simulink subsystem "LRLM_ECU"  (R2021a)
settings: Solver=VariableStepAuto  StartTime=0.0  StopTime=10.0  RelTol=1e-3
values from neighbouring files (symbols this model uses):
  op_type = 2    [baseworkspace_variables.mat]
libraries: LRLM x4, simulink x2, pil_lib x1, BCM x1
settings Model: Creator=Sai229  LastModifiedBy=Sai229

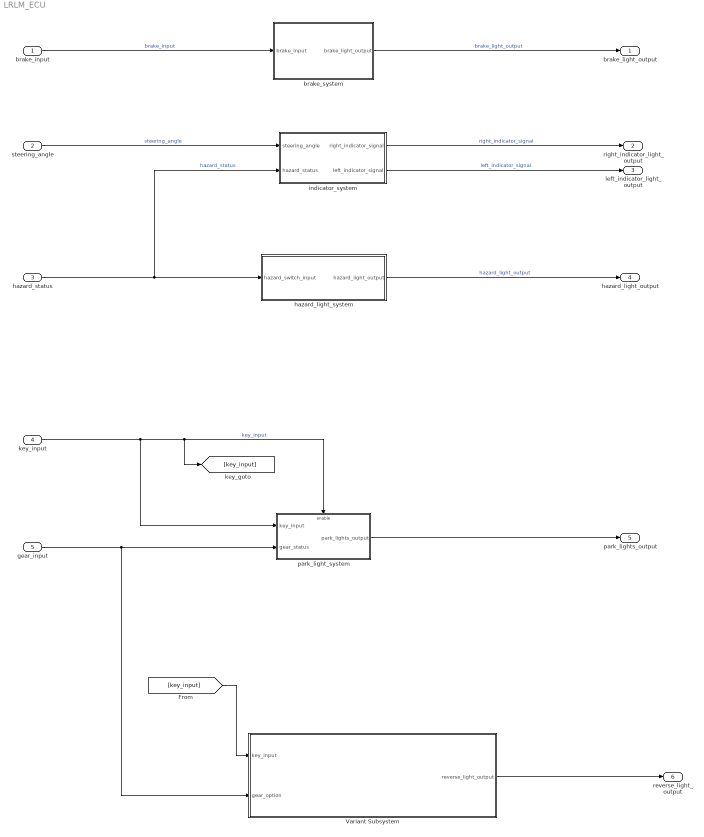
== system LRLM_ECU ==
  brake_input : Inport
  steering_angle : Inport  Port=2
  hazard_status : Inport  Port=3
  key_input : Inport  Port=4
  gear_input : Inport  Port=5
  Variant Subsystem : Subsystem  Variant=on
  brake_system : Subsystem  TreatAsAtomicUnit=on
      mask Display: disp("Brake System");
  hazard_light_system : Subsystem
  indicator_system : Subsystem  TreatAsAtomicUnit=on
  park_light_system : Subsystem
  brake_light_output : Outport
  right_indicator_light_output : Outport  Port=2
  left_indicator_light_output : Outport  Port=3
  hazard_light_output : Outport  Port=4
  park_lights_output : Outport  Port=5
  reverse_light_output : Outport  Port=6
  wires:
  hazard_light_system/1(hazard_light_output) -> hazard_light_output/1  "hazard_light_output"
  brake_input/1 -> brake_system/1(brake_input)  "brake_input"
  park_light_system/1(park_lights_output) -> park_lights_output/1
  key_input/1 -> park_light_system/Enable, [key_input], park_light_system/1(key_input)  "key_input"
  hazard_status/1 -> hazard_light_system/1(hazard_switch_input), indicator_system/2(hazard_status)  "hazard_status"
  indicator_system/2(left_indicator_signal) -> left_indicator_light_output/1  "left_indicator_signal"
  indicator_system/1(right_indicator_signal) -> right_indicator_light_output/1  "right_indicator_signal"
  steering_angle/1 -> indicator_system/1(steering_angle)  "steering_angle"
  brake_system/1(brake_light_output) -> brake_light_output/1  "brake_light_output"
  gear_input/1 -> park_light_system/2(gear_status), Variant Subsystem/2(gear_option)
  [key_input] -> Variant Subsystem/1(key_input)
  Variant Subsystem/1(reverse_light_output) -> reverse_light_output/1

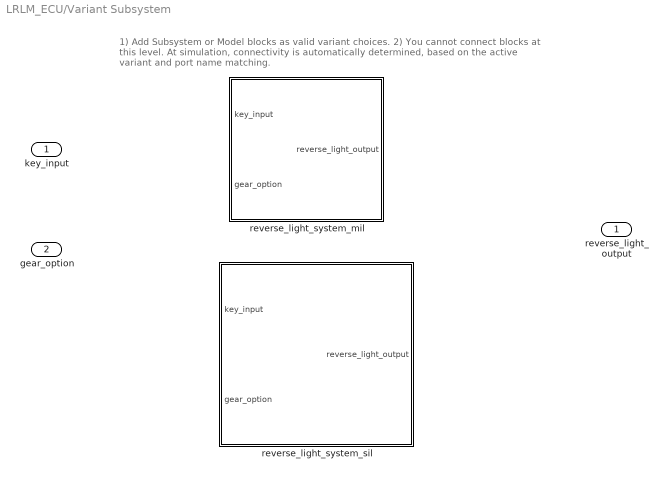
== system LRLM_ECU/Variant Subsystem ==
  note: 1) Add Subsystem or Model blocks as valid variant choices.
      | 2) You cannot connect blocks at this level. At simulation, connectivity is automatically
      | determined, based on the active variant and port name matching.
  key_input : Inport
  gear_option : Inport  Port=2
  reverse_light_system_mil : Subsystem  TreatAsAtomicUnit=on  VariantControl=reverse_light_sys_sil  mask{out_type=Reverse Lights will not Blink}
      mask prompts: out_type "Output type"
      mask init:
      | assignin('base','op_type',out_type);
      mask TypeOptions out_type: Reverse Lights will Blink | Reverse Lights will not Blink
  reverse_light_system_sil : Subsystem  DialogController=pil_create_dialog  LoadFcn=|  VariantControl=reverse_light_sys_mil
      | try
      |    if ~strcmp(rtw.pil.getPILVersion, '9.10 (R2021a)_15')
      |       set_param(gcb, 'DialogController', '');
      |       set_param(gcb, 'DialogControllerArgs', '');
      |    end
      | catch e
      |       set_param(gcb, 'DialogController', '');
      |       set_param(gcb, 'DialogControllerArgs', '');
      | end
      mask help: PIL:pil:XILBlockMaskDesc
      mask Display: disp('SIL');
  reverse_light_output : Outport

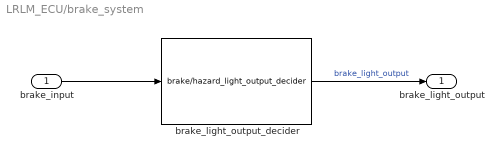
== system LRLM_ECU/brake_system ==
  brake_input : Inport
  brake_light_output_decider : LRLM/brake//hazard_light_output_decider
      settings: SourceProductName=LRLM Library
  brake_light_output : Outport
  wires:
  brake_light_output_decider/1 -> brake_light_output/1  "brake_light_output"
  brake_input/1 -> brake_light_output_decider/1

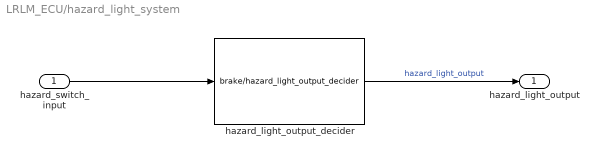
== system LRLM_ECU/hazard_light_system ==
  hazard_switch_input : Inport
  hazard_light_output_decider : LRLM/brake//hazard_light_output_decider
      settings: SourceProductName=LRLM Library
  hazard_light_output : Outport
  wires:
  hazard_light_output_decider/1 -> hazard_light_output/1  "hazard_light_output"
  hazard_switch_input/1 -> hazard_light_output_decider/1

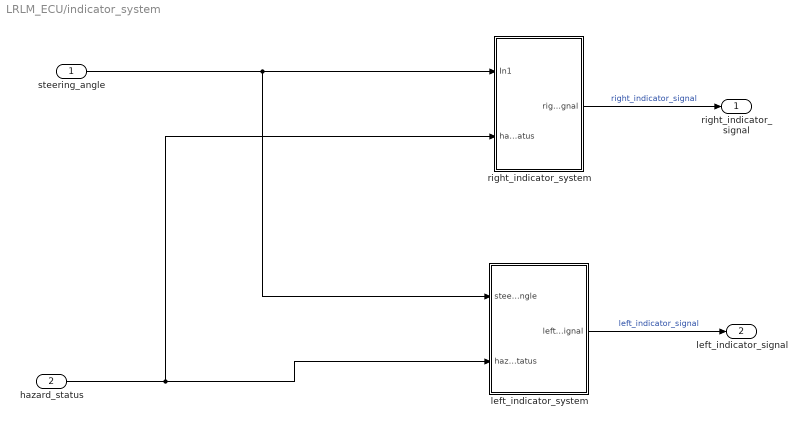
== system LRLM_ECU/indicator_system ==
  steering_angle : Inport
  hazard_status : Inport  Port=2
  left_indicator_system : Subsystem
  right_indicator_system : Subsystem
  right_indicator_signal : Outport
  left_indicator_signal : Outport  Port=2
  wires:
  steering_angle/1 -> right_indicator_system/1(In1), left_indicator_system/1(steering_angle)
  hazard_status/1 -> left_indicator_system/2(hazard_status), right_indicator_system/2(hazard_status)
  right_indicator_system/1(right_indicator_signal) -> right_indicator_signal/1  "right_indicator_signal"
  left_indicator_system/1(left_indicator_signal) -> left_indicator_signal/1  "left_indicator_signal"

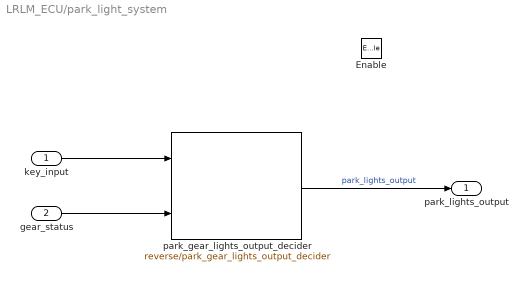
== system LRLM_ECU/park_light_system ==
  key_input : Inport
  gear_status : Inport  Port=2
  Enable : EnablePort  StatesWhenEnabling=reset
  park_gear_lights_output_decider : BCM/reverse//park_gear_lights_output_decider  gear_option=Park
      settings: SourceProductName=BCM Library
  park_lights_output : Outport
  wires:
  park_gear_lights_output_decider/1 -> park_lights_output/1  "park_lights_output"
  gear_status/1 -> park_gear_lights_output_decider/2
  key_input/1 -> park_gear_lights_output_decider/1

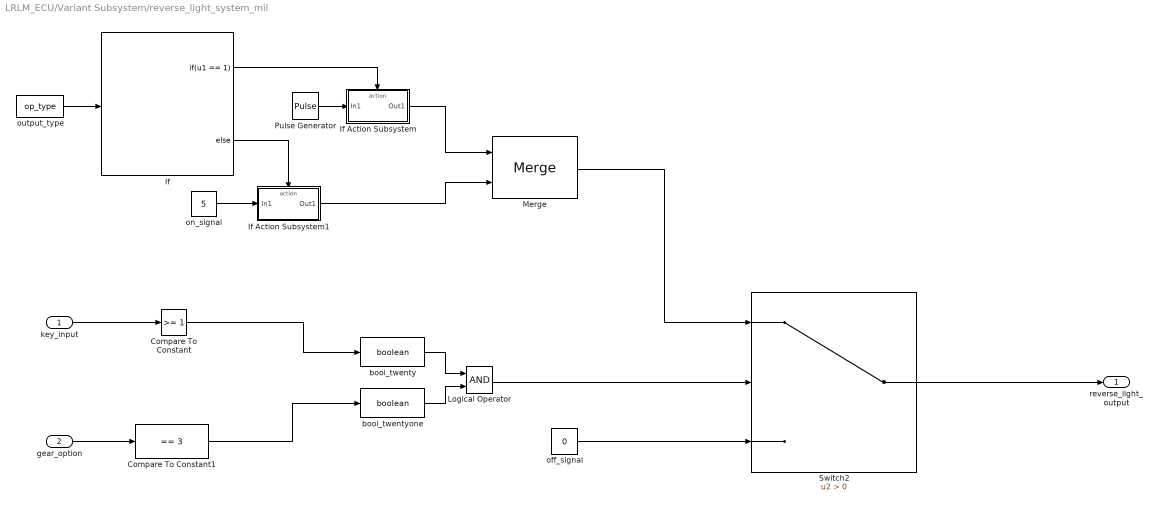
== system LRLM_ECU/Variant Subsystem/reverse_light_system_mil ==
  key_input : Inport
  gear_option : Inport  Port=2
  Compare To Constant : simulink/Logic and Bit Operations/Compare To Constant  relop=>=  const=1  OutDataTypeStr=boolean
  Compare To Constant1 : simulink/Logic and Bit Operations/Compare To Constant  relop===  const=3  OutDataTypeStr=boolean
  If : If  IfExpression=u1 == 1
  If Action Subsystem : Subsystem  TreatAsAtomicUnit=on
  If Action Subsystem1 : Subsystem  TreatAsAtomicUnit=on
  Logical Operator : Logic  AllPortsSameDT=off  OutDataTypeStr=boolean
  Merge : Merge
  Pulse Generator : DiscretePulseGenerator  PulseType=Time based  Amplitude=5  Period=0.1  PulseWidth=5
  Switch2 : Switch  Criteria=u2 > Threshold
  bool_twenty : DataTypeConversion  OutDataTypeStr=boolean
  bool_twentyone : DataTypeConversion  OutDataTypeStr=boolean
  off_signal : Constant  Value=0
  on_signal : Constant  Value=5
  output_type : Constant  Value=op_type
  reverse_light_output : Outport
  wires:
  Switch2/1 -> reverse_light_output/1
  output_type/1 -> If/1
  on_signal/1 -> If Action Subsystem1/1(In1)
  Pulse Generator/1 -> If Action Subsystem/1(In1)
  If/2 -> If Action Subsystem1/Action
  If Action Subsystem1/1(Out1) -> Merge/2
  If/1 -> If Action Subsystem/Action
  If Action Subsystem/1(Out1) -> Merge/1
  key_input/1 -> Compare To Constant/1
  gear_option/1 -> Compare To Constant1/1
  Compare To Constant1/1 -> bool_twentyone/1
  Compare To Constant/1 -> bool_twenty/1
  bool_twenty/1 -> Logical Operator/1
  Merge/1 -> Switch2/1
  off_signal/1 -> Switch2/3
  bool_twentyone/1 -> Logical Operator/2
  Logical Operator/1 -> Switch2/2

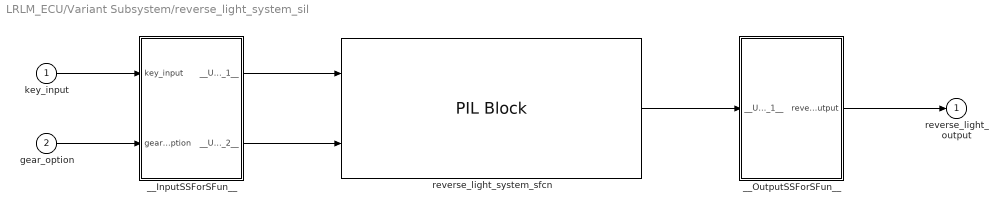
== system LRLM_ECU/Variant Subsystem/reverse_light_system_sil ==
  key_input : Inport
  gear_option : Inport  Port=2
  __InputSSForSFun__ : Subsystem
  __OutputSSForSFun__ : Subsystem
  reverse_light_system_sfcn : pil_lib/PIL Block  SimulationMode=SIL  IsTopModelPIL=off  CodeDir=D:\Genesis\HILClimbers_Public_Project\reverse_light_system_ert_rtw  AnchorDir=D:\Genesis\HILClimbers_Public_Project  ConfigName=Software-in-the-Loop (SIL)  XrelIsTopModelCode=on  XrelIsReusable=off  XrelDWorkNames={}  XrelDWorkTypes={}  XrelModelArgVals={}  XrelOrderedParamNames={}
      settings: SourceProductBaseCode=RT
  reverse_light_output : Outport
  wires:
  __OutputSSForSFun__/1(reverse_light_output) -> reverse_light_output/1
  reverse_light_system_sfcn/1 -> __OutputSSForSFun__/1(__UniqueInportName__1__)
  __InputSSForSFun__/2(__UniqueOutportName__2__) -> reverse_light_system_sfcn/2
  __InputSSForSFun__/1(__UniqueOutportName__1__) -> reverse_light_system_sfcn/1
  gear_option/1 -> __InputSSForSFun__/2(gear_option)
  key_input/1 -> __InputSSForSFun__/1(key_input)

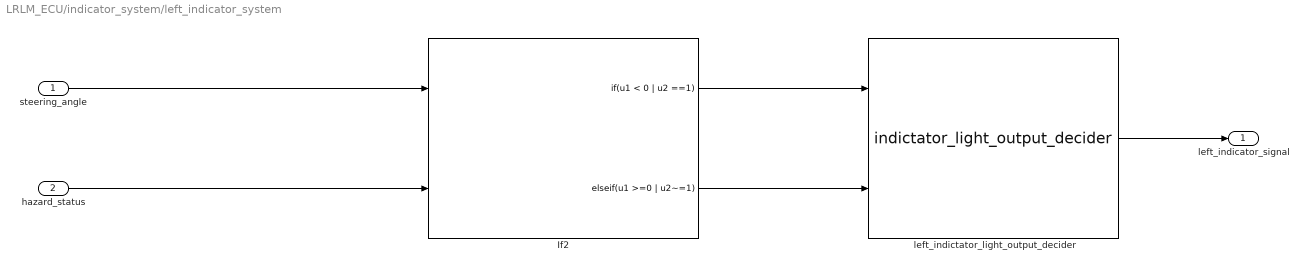
== system LRLM_ECU/indicator_system/left_indicator_system ==
  steering_angle : Inport
  hazard_status : Inport  Port=2
  If2 : If  NumInputs=2  IfExpression=u1 < 0 | u2 ==1  ElseIfExpressions=u1 >=0 | u2~=1  ShowElse=off
  left_indictator_light_output_decider : LRLM/indictator_light_output_decider
      settings: SourceProductName=LRLM Library
  left_indicator_signal : Outport
  wires:
  left_indictator_light_output_decider/1 -> left_indicator_signal/1
  If2/2 -> left_indictator_light_output_decider/2
  If2/1 -> left_indictator_light_output_decider/1
  steering_angle/1 -> If2/1
  hazard_status/1 -> If2/2

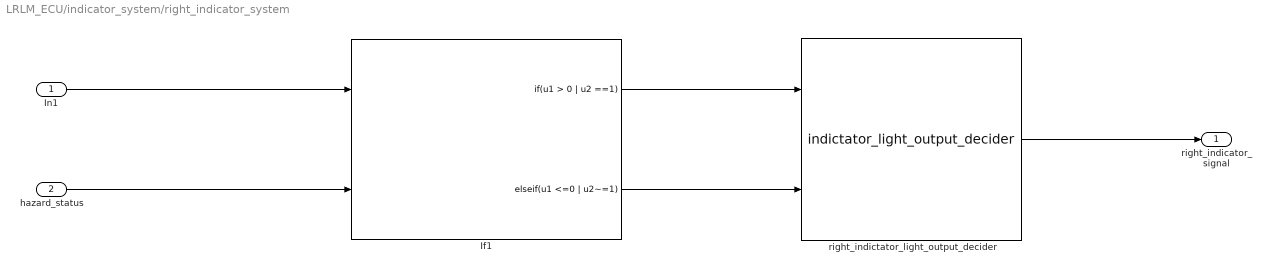
== system LRLM_ECU/indicator_system/right_indicator_system ==
  In1 : Inport
  hazard_status : Inport  Port=2
  If1 : If  NumInputs=2  IfExpression=u1 > 0 | u2 ==1  ElseIfExpressions=u1 <=0 | u2~=1  ShowElse=off
  right_indictator_light_output_decider : LRLM/indictator_light_output_decider
      settings: SourceProductName=LRLM Library
  right_indicator_signal : Outport
  wires:
  right_indictator_light_output_decider/1 -> right_indicator_signal/1
  If1/2 -> right_indictator_light_output_decider/2
  If1/1 -> right_indictator_light_output_decider/1
  In1/1 -> If1/1
  hazard_status/1 -> If1/2

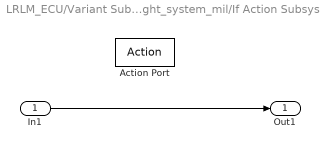
== system LRLM_ECU/Variant Subsystem/reverse_light_system_mil/If Action Subsystem ==
  In1 : Inport
  Action Port : ActionPort
  Out1 : Outport
  wires:
  In1/1 -> Out1/1

== system LRLM_ECU/Variant Subsystem/reverse_light_system_mil/If Action Subsystem1 ==
  In1 : Inport
  Action Port : ActionPort
  Out1 : Outport
  wires:
  In1/1 -> Out1/1

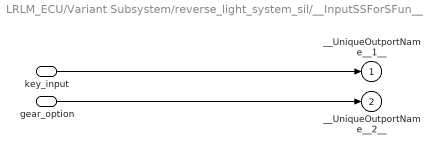
== system LRLM_ECU/Variant Subsystem/reverse_light_system_sil/__InputSSForSFun__ ==
  key_input : Inport
  gear_option : Inport  Port=2
  __UniqueOutportName__1__ : Outport
  __UniqueOutportName__2__ : Outport  Port=2
  wires:
  gear_option/1 -> __UniqueOutportName__2__/1
  key_input/1 -> __UniqueOutportName__1__/1

== system LRLM_ECU/Variant Subsystem/reverse_light_system_sil/__OutputSSForSFun__ ==
  __UniqueInportName__1__ : Inport
  reverse_light_output : Outport
  wires:
  __UniqueInportName__1__/1 -> reverse_light_output/1
